simulink model "visualize_2019a"  (R2022a)
settings: Solver=VariableStepAuto  StartTime=0.0  StopTime=inf  RelTol=1e-3
undefined symbols (not defined in the file or in its folder): A, b, NULL
libraries: instrumentseriallib x2
settings Model: Creator=alvin  LastModifiedBy=alvin
settings SolverCC: AlgebraicLoopSolver=TrustRegion
settings DebuggingCC: UnconnectedInputMsg=warning  UnconnectedOutputMsg=warning  UnconnectedLineMsg=warning  SFMachineParentedDataDiag=warning
settings SFSimCC: CustomCodeUndefinedFunction=UseInterfaceOnly

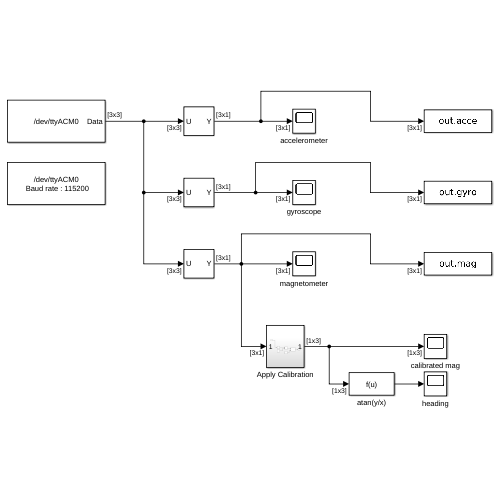
[thumbnail: Simulink's stored preview of the top-level diagram]
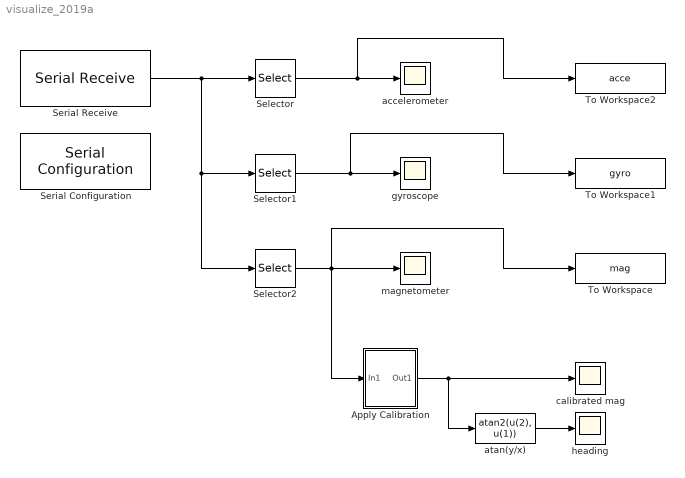
== system visualize_2019a ==
  Apply Calibration : Subsystem  LoadFcn=|
      | A = eye(3);
      | b = [0 0 0];
  Selector : Selector  NumberOfDimensions=2  InputPortWidth=3  IndexOptions=Select all,Index vector (dialog)  Indices=[1 3],1  OutputSizes=1,1
  Selector1 : Selector  NumberOfDimensions=2  InputPortWidth=3  IndexOptions=Select all,Index vector (dialog)  Indices=[1 3],2  OutputSizes=1,1
  Selector2 : Selector  NumberOfDimensions=2  InputPortWidth=3  IndexOptions=Select all,Index vector (dialog)  Indices=[1 3],3  OutputSizes=1,1
  Serial Configuration : instrumentseriallib/Serial Configuration  Priority=-200000  PortSel=/dev/ttyACM0  Port=/dev/ttyACM0  ComPort=/dev/ttyACM0  BaudRate=115200  DataBits=8  Parity=none  StopBits=1  ByteOrder=little-endian  FlowControl=none  Timeout=10  SimulateUsing=Interpreted execution  BlockInModel=on  aMode=1
      settings: SourceProductBaseCode=OT,IC,MT
  Serial Receive : instrumentseriallib/Serial Receive  PortSel=/dev/ttyACM0  Port=/dev/ttyACM0  ComPort=/dev/ttyACM0  DataType=single  SaveDataType=uint8  ToggleHeader=on  Header=[ 115 ]  ToggleTerminator=on  Terminator=NULL ('\0')  CustomTerminator=[]  InputFormat=Column major  ToggleDataSize=on  DataSize="[3  3]"  EnableBlockingMode=on  ActionDataUnavailable=Output last received value  ActionWhenDataUnavailable=Output last received value  CustomValue=0  SampleTime=0.01  SimulateUsing=Interpreted execution  BlockInModel=on  aMode=1
      settings: SourceProductBaseCode=OT,IC,MT
  To Workspace : ToWorkspace  VariableName=mag  SampleTime=-1
  To Workspace1 : ToWorkspace  VariableName=gyro  SampleTime=-1
  To Workspace2 : ToWorkspace  VariableName=acce  SampleTime=-1
  accelerometer : Scope
  atan(y/x) : Fcn  Expr=atan2(u(2), u(1))
  calibrated mag : Scope
  gyroscope : Scope
  heading : Scope
  magnetometer : Scope
  wires:
  Selector/1 -> To Workspace2/1, accelerometer/1
  Selector1/1 -> To Workspace1/1, gyroscope/1
  Selector2/1 -> Apply Calibration/1(In1), To Workspace/1, magnetometer/1
  Serial Receive/1 -> Selector1/1, Selector2/1, Selector/1
  atan(y/x)/1 -> heading/1
  Apply Calibration/1(Out1) -> atan(y/x)/1, calibrated mag/1

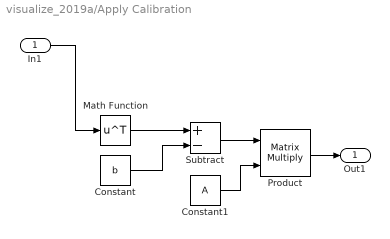
== system visualize_2019a/Apply Calibration ==
  In1 : Inport
  Constant : Constant  Value=b  VectorParams1D=off
  Constant1 : Constant  Value=A  VectorParams1D=off
  Math Function : Math  Operator=transpose  SignedPower=on
  Product : Product  Multiplication=Matrix(*)
  Subtract : Sum  Inputs=+-
  Out1 : Outport
  wires:
  Constant/1 -> Subtract/2
  Math Function/1 -> Subtract/1
  In1/1 -> Math Function/1
  Product/1 -> Out1/1
  Subtract/1 -> Product/1
  Constant1/1 -> Product/2
